simulink model "HDLTx"  (R2024a)
settings: Solver=FixedStepDiscrete  StartTime=0.0  StopTime=stopTime  RelTol=1e-3
values from neighbouring files (symbols this model uses):
  msgIn = cell(1,1); msgIn{1} = a    [tx.m]
  pWords = [pWords binl2str(pBits{i})]    [tx.m]
undefined symbols (not defined in the file or in its folder): CONST
libraries: dspsrcs4 x6, simulink x4, hdlsllib x4, whdlutilities x2, HDL_ieee_8021513 x2
settings Model: DataTypeOverride=Off  SimulationMode=accelerator  Creator=cotti  LastModifiedBy=cotti
settings OptimizationCC: BlockReduction=off  ConditionallyExecuteInputs=off  DefaultParameterBehavior=Inlined  InheritOutputTypeSmallerThanSingle=on  ReuseModelBlockBuffer=off
settings DebuggingCC: AlgebraicLoopMsg=error  SingleTaskRateTransMsg=error  UnconnectedInputMsg=warning  UnconnectedOutputMsg=warning  UnconnectedLineMsg=warning
settings HardwareCC: ProdBitPerPointer=32  ProdBitPerSizeT=32  ProdBitPerPtrDiffT=32  ProdLargestAtomicFloat=None  ProdIntDivRoundTo=Undefined  ProdEndianess=Unspecified  ProdWordSize=32  ProdHWDeviceType=ASIC/FPGA->ASIC/FPGA  TargetBitPerLong=64  TargetBitPerPointer=64  TargetBitPerSizeT=64  TargetBitPerPtrDiffT=64  TargetLongLongMode=on  TargetIntDivRoundTo=Zero  TargetEndianess=LittleEndian  TargetWordSize=64  TargetHWDeviceType=Custom Processor->MATLAB Host Computer  ProdEqTarget=off
settings RTWCC: GPUComputeCapability=3.5

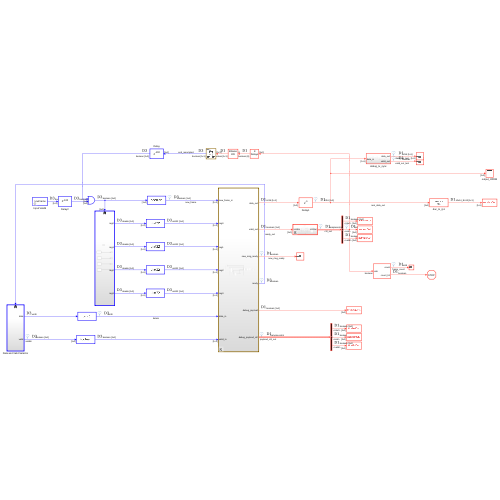
[thumbnail: Simulink's stored preview of the top-level diagram]
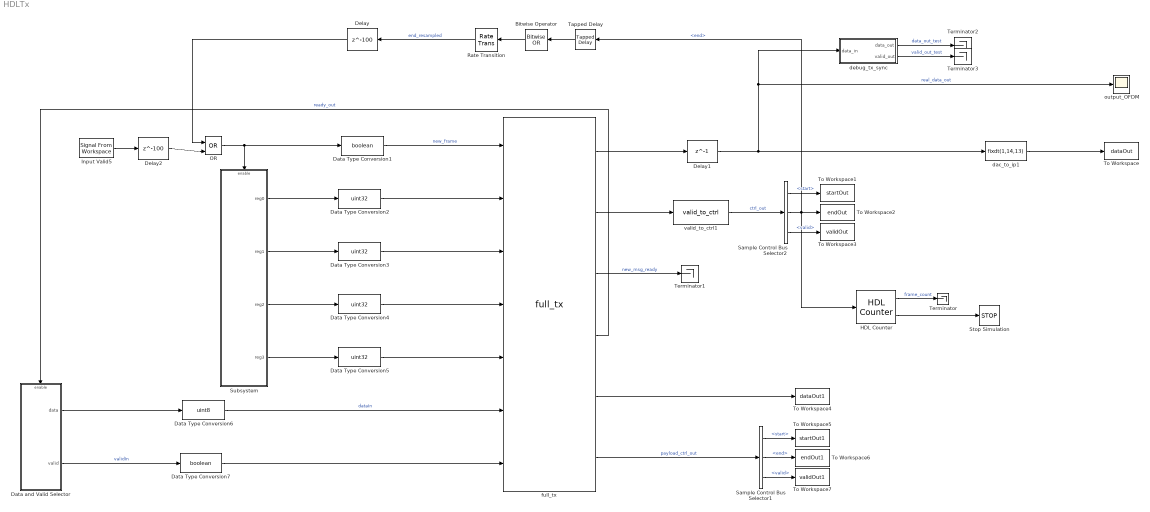
== system HDLTx ==
  Bitwise Operator : simulink/Logic and Bit Operations/Bitwise Operator  logicop=OR  UseBitMask=off  BitMask=bin2dec('11011001')  BitMaskRealWorld=Stored Integer
      settings: LibrarySourceBlock=|
      | hdlsllib/Logic and Bit
      | Operations/Bitwise
      | Operator
  Data Type Conversion1 : DataTypeConversion  OutDataTypeStr=boolean  SaturateOnIntegerOverflow=off  RndMeth=Floor
  Data Type Conversion{2..5} (4 alike) : DataTypeConversion  OutDataTypeStr=uint32  SaturateOnIntegerOverflow=off  RndMeth=Floor
  Data Type Conversion6 : DataTypeConversion  OutDataTypeStr=uint8  SaturateOnIntegerOverflow=off  RndMeth=Floor
  Data Type Conversion7 : DataTypeConversion  OutDataTypeStr=boolean  SaturateOnIntegerOverflow=off  RndMeth=Floor
  Data and Valid Selector : Subsystem  TreatAsAtomicUnit=on
  Delay : Delay  DelayLength=100  InitialCondition=0  UseCircularBuffer=on
  Delay1 : Delay  DelayLength=1  InitialCondition=0  UseCircularBuffer=on
  Delay2 : Delay  DelayLength=100  InitialCondition=0  UseCircularBuffer=on
  HDL Counter : hdlsllib/Sources/HDL Counter  CountType=Count limited  CountInit=0  CountStep=1  CountMax=length(msgIn)  CountFromType=Initial value  CountFrom=0  CountResetPort=off  CountLoadPort=off  CountEnbPort=on  CountDirPort=off  CountHitOutputPort=on  CountDataType=Unsigned  CountWordLen=8  CountFracLen=0  CountSampTime=1
  Input Valid5 : dspsrcs4/Signal From Workspace  X=newFrame  Ts=4/CONST.fPHY  nsamps=1  OutputAfterFinalValue=Setting to zero  ignoreOrWarnInputAndFrameLengths=off  OutputFrames=off
  OR : Logic  Operator=OR  IconShape=distinctive  AllPortsSameDT=off  OutDataTypeStr=boolean
  Rate Transition : RateTransition  OutPortSampleTime=4/CONST.fPHY
  Sample Control Bus Selector1 : whdlutilities/Sample Control Bus Selector  OutputSignals=start,end,valid
  Sample Control Bus Selector2 : whdlutilities/Sample Control Bus Selector  OutputSignals=start,end,valid
  Stop Simulation : Stop
  Subsystem : Subsystem
  Tapped Delay : simulink/Discrete/Tapped Delay  vinit=0.0  samptime=-1  NumDelays=8  DelayOrder=Oldest  includeCurrent=off
  Terminator{,1..3} (4 alike) : Terminator
  To Workspace : ToWorkspace  VariableName=dataOut  SampleTime=1/CONST.fDAC
      settings: Save2DSignal=2-D array (concatenate along first dimension)
  To Workspace1 : ToWorkspace  VariableName=startOut  SampleTime=1/CONST.fDAC
      settings: Save2DSignal=2-D array (concatenate along first dimension)
  To Workspace2 : ToWorkspace  VariableName=endOut  SampleTime=1/CONST.fDAC
      settings: Save2DSignal=2-D array (concatenate along first dimension)
  To Workspace3 : ToWorkspace  VariableName=validOut  SampleTime=1/CONST.fDAC
      settings: Save2DSignal=2-D array (concatenate along first dimension)
  To Workspace4 : ToWorkspace  VariableName=dataOut1  SampleTime=1/CONST.fs
      settings: Save2DSignal=2-D array (concatenate along first dimension)
  To Workspace5 : ToWorkspace  VariableName=startOut1  SampleTime=1/CONST.fs
      settings: Save2DSignal=2-D array (concatenate along first dimension)
  To Workspace6 : ToWorkspace  VariableName=endOut1  SampleTime=1/CONST.fs
      settings: Save2DSignal=2-D array (concatenate along first dimension)
  To Workspace7 : ToWorkspace  VariableName=validOut1  SampleTime=1/CONST.fs
      settings: Save2DSignal=2-D array (concatenate along first dimension)
  dac_to_ip1 : DataTypeConversion  OutDataTypeStr=fixdt(1,14,13)  ConvertRealWorld=Stored Integer (SI)  SaturateOnIntegerOverflow=off  RndMeth=Floor
  debug_tx_sync : Subsystem
  full_tx : HDL_ieee_8021513/full_tx  SystemSampleTime=-1  VariantActivationTime=update diagram  AllowFlexibleInterface=on  Latency=0  AutoFrameSizeCalculation=off
      settings: SourceProductName=HDL IEEE 8021513
  output_OFDM : Scope
  valid_to_ctrl1 : HDL_ieee_8021513/valid_to_ctrl  SystemSampleTime=-1  VariantActivationTime=update diagram  AllowFlexibleInterface=on  Latency=0  AutoFrameSizeCalculation=off
      settings: SourceProductName=HDL IEEE 8021513
  wires:
  Sample Control Bus Selector2/1 -> To Workspace1/1  "<start>"
  Sample Control Bus Selector2/2 -> Tapped Delay/1, HDL Counter/1, To Workspace2/1  "<end>"
  Sample Control Bus Selector2/3 -> To Workspace3/1  "<valid>"
  valid_to_ctrl1/1 -> Sample Control Bus Selector2/1  "ctrl_out"
  Delay1/1 -> dac_to_ip1/1, debug_tx_sync/1(data_in), output_OFDM/1  "real_data_out"
  Data and Valid Selector/1(data) -> Data Type Conversion6/1
  Data and Valid Selector/2(valid) -> Data Type Conversion7/1  "validIn"
  Data Type Conversion1/1 -> full_tx/1  "new_frame"
  Data Type Conversion2/1 -> full_tx/2
  Data Type Conversion3/1 -> full_tx/3
  Data Type Conversion4/1 -> full_tx/4
  Data Type Conversion5/1 -> full_tx/5
  Data Type Conversion6/1 -> full_tx/6  "dataIn"
  full_tx/1 -> Delay1/1
  full_tx/2 -> valid_to_ctrl1/1
  full_tx/4 -> Data and Valid Selector/Enable  "ready_out"
  Sample Control Bus Selector1/1 -> To Workspace5/1  "<start>"
  full_tx/6 -> Sample Control Bus Selector1/1  "payload_ctrl_out"
  Sample Control Bus Selector1/3 -> To Workspace7/1  "<valid>"
  Sample Control Bus Selector1/2 -> To Workspace6/1  "<end>"
  full_tx/5 -> To Workspace4/1
  OR/1 -> Subsystem/Enable, Data Type Conversion1/1
  Input Valid5/1 -> Delay2/1
  HDL Counter/1 -> Terminator/1  "frame_count"
  HDL Counter/2 -> Stop Simulation/1
  Rate Transition/1 -> Delay/1  "end_resampled"
  Tapped Delay/1 -> Bitwise Operator/1
  Bitwise Operator/1 -> Rate Transition/1
  Subsystem/1(reg0) -> Data Type Conversion2/1
  Subsystem/2(reg1) -> Data Type Conversion3/1
  Subsystem/3(reg2) -> Data Type Conversion4/1
  Subsystem/4(reg3) -> Data Type Conversion5/1
  Data Type Conversion7/1 -> full_tx/7
  full_tx/3 -> Terminator1/1  "new_msg_ready"
  Delay/1 -> OR/1
  dac_to_ip1/1 -> To Workspace/1
  Delay2/1 -> OR/2
  debug_tx_sync/1(data_out) -> Terminator2/1  "data_out_test"
  debug_tx_sync/2(valid_out) -> Terminator3/1  "valid_out_test"

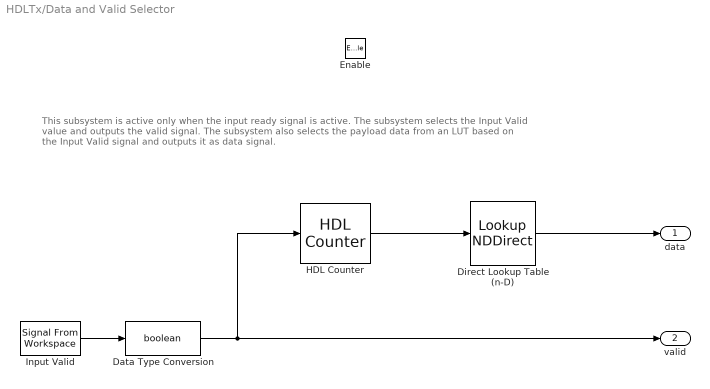
== system HDLTx/Data and Valid Selector ==
  note: This subsystem is active only when the input ready signal is active. The subsystem selects the Input Valid value and outputs the valid signal.
      | The subsystem also selects the payload data from an LUT based on the Input Valid signal and outputs it as data signal.
  Enable : EnablePort
  Data Type Conversion : DataTypeConversion  OutDataTypeStr=boolean  SaturateOnIntegerOverflow=off  RndMeth=Floor
  Direct Lookup Table (n-D) : LookupNDDirect  NumberOfTableDimensions=1  Table=uint8(pWords')  DiagnosticForOutOfRangeInput=Error  TableDataTypeStr=uint8
  HDL Counter : hdlsllib/Sources/HDL Counter  CountType=Count limited  CountInit=0  CountStep=1  CountMax=length(pWords) -1  CountFromType=Initial value  CountFrom=0  CountResetPort=off  CountLoadPort=off  CountEnbPort=on  CountDirPort=off  CountHitOutputPort=off  CountDataType=Unsigned  CountWordLen=nextpow2(length(pWords))  CountFracLen=0  CountSampTime=1
  Input Valid : dspsrcs4/Signal From Workspace  X=validIn  Ts=4/CONST.fPHY  nsamps=1  OutputAfterFinalValue=Setting to zero  ignoreOrWarnInputAndFrameLengths=off  OutputFrames=off
  data : Outport  InitialOutput=0  VectorParamsAs1DForOutWhenUnconnected=off
  valid : Outport  Port=2  InitialOutput=0  VectorParamsAs1DForOutWhenUnconnected=off
  wires:
  HDL Counter/1 -> Direct Lookup Table (n-D)/1
  Direct Lookup Table (n-D)/1 -> data/1
  Input Valid/1 -> Data Type Conversion/1
  Data Type Conversion/1 -> valid/1, HDL Counter/1

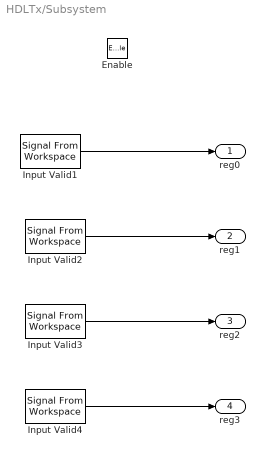
== system HDLTx/Subsystem ==
  Enable : EnablePort
  Input Valid1 : dspsrcs4/Signal From Workspace  X=reg0  Ts=4/CONST.fPHY  nsamps=1  OutputAfterFinalValue=Setting to zero  ignoreOrWarnInputAndFrameLengths=off  OutputFrames=off
  Input Valid2 : dspsrcs4/Signal From Workspace  X=reg1  Ts=4/CONST.fPHY  nsamps=1  OutputAfterFinalValue=Setting to zero  ignoreOrWarnInputAndFrameLengths=off  OutputFrames=off
  Input Valid3 : dspsrcs4/Signal From Workspace  X=reg2  Ts=4/CONST.fPHY  nsamps=1  OutputAfterFinalValue=Setting to zero  ignoreOrWarnInputAndFrameLengths=off  OutputFrames=off
  Input Valid4 : dspsrcs4/Signal From Workspace  X=reg3  Ts=4/CONST.fPHY  nsamps=1  OutputAfterFinalValue=Setting to zero  ignoreOrWarnInputAndFrameLengths=off  OutputFrames=off
  reg0 : Outport
  reg1 : Outport  Port=2
  reg2 : Outport  Port=3
  reg3 : Outport  Port=4
  wires:
  Input Valid4/1 -> reg3/1
  Input Valid2/1 -> reg1/1
  Input Valid1/1 -> reg0/1
  Input Valid3/1 -> reg2/1

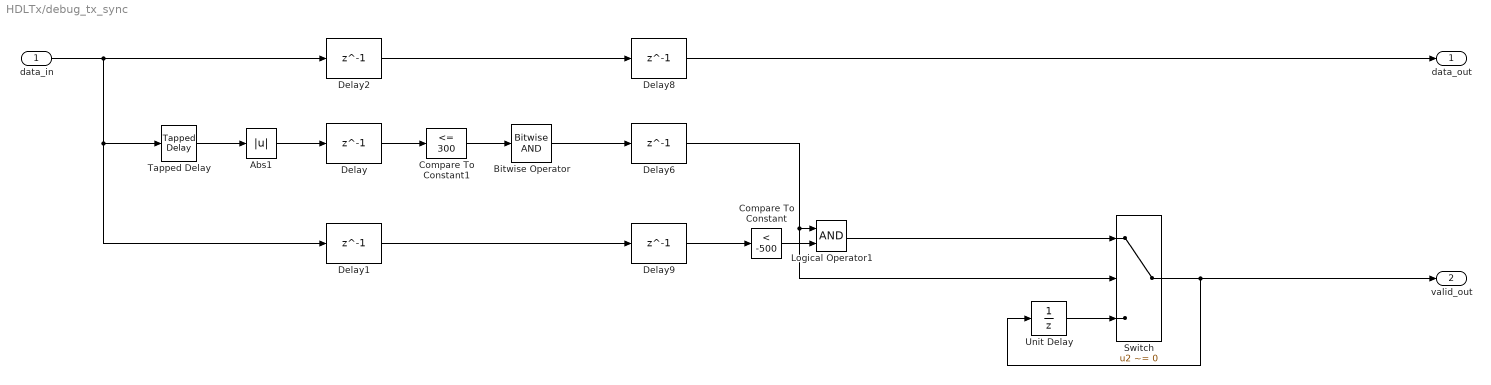
== system HDLTx/debug_tx_sync ==
  data_in : Inport
  Abs1 : Abs  SaturateOnIntegerOverflow=off
  Bitwise Operator : simulink/Logic and Bit Operations/Bitwise Operator  logicop=AND  UseBitMask=off  BitMask=bin2dec('11011001')  BitMaskRealWorld=Stored Integer
      settings: LibrarySourceBlock=|
      | hdlsllib/Logic and Bit
      | Operations/Bitwise
      | Operator
  Compare To Constant : hdlsllib/Logic and Bit Operations/Compare To Constant  relop=<  const=-500  OutDataTypeStr=boolean
  Compare To Constant1 : hdlsllib/Logic and Bit Operations/Compare To Constant  relop=<=  const=300  OutDataTypeStr=boolean
  Delay{,1..2,6,8..9} (6 alike) : Delay  DelayLength=1  InitialCondition=0  UseCircularBuffer=on
  Logical Operator1 : Logic  AllPortsSameDT=off  OutDataTypeStr=boolean
  Switch : Switch  Criteria=u2 ~= 0  SaturateOnIntegerOverflow=off  InputSameDT=off
  Tapped Delay : simulink/Discrete/Tapped Delay  vinit=0.0  samptime=-1  NumDelays=8  DelayOrder=Oldest  includeCurrent=off
      settings: LibrarySourceBlock=hdlsllib/Discrete/Tapped Delay
  Unit Delay : UnitDelay  SampleTime=-1  HasFrameUpgradeWarning=on
  data_out : Outport
  valid_out : Outport  Port=2
  wires:
  Tapped Delay/1 -> Abs1/1
  Abs1/1 -> Delay/1
  Switch/1 -> Unit Delay/1, valid_out/1
  Delay/1 -> Compare To Constant1/1
  Logical Operator1/1 -> Switch/1
  Unit Delay/1 -> Switch/3
  Bitwise Operator/1 -> Delay6/1
  data_in/1 -> Delay2/1, Delay1/1, Tapped Delay/1
  Compare To Constant/1 -> Logical Operator1/2
  Compare To Constant1/1 -> Bitwise Operator/1
  Delay1/1 -> Delay9/1
  Delay2/1 -> Delay8/1
  Delay6/1 -> Switch/2, Logical Operator1/1
  Delay8/1 -> data_out/1
  Delay9/1 -> Compare To Constant/1
